simulink model "uz_ParameterID6ph"  (R2021b)
settings: Solver=FixedStepDiscrete  StartTime=0.0  StopTime=160  FixedStep=0.000005  RelTol=1e-3  EnableMultiTasking=on
model workspace (MATLAB code in the model file):
  | cmdLim = Simulink.Parameter;
  | cmdLim.Value = 15;
  | cmdLim.Description = 'Limit for controlling the maximum surface command angle.';
  | cmdLim.Min = 0;
  | cmdLim.Max = 90;
  | cmdLim.DocUnits = 'deg';
  | 
  | dispGain = Simulink.Parameter;
  | dispGain.Value = 0.75;
  | dispGain.Description = 'Gain applied to the displacement error.';
  | dispGain.Min = 0;
  | dispGain.Max = [];
  | dispGain.DocUnits = 'deg/sec/deg';
  | 
  | dispLim = Simulink.Parameter;
  | dispLim.Value = 30;
  | dispLim.Description = 'Limit for controlling the maximum commanded angle.';
  | dispLim.Min = 0;
  | dispLim.Max = 180;
  | dispLim.DocUnits = 'deg';
  | 
  | intGain = Simulink.Parameter;
  | intGain.Value = 0.5;
  | intGain.Description = 'Gain applied to the integral error.';
  | intGain.Min = 0;
  | intGain.Max = [];
  | intGain.DocUnits = 'deg/sec/deg/sec';
  | 
  | intLim = Simulink.Parameter;
  | intLim.Value = 5;
  | intLim.Description = 'Limit for controlling the maximum commanded angle.';
  | intLim.Min = 0;
  | intLim.Max = 90;
  | intLim.DocUnits = 'deg';
  | 
  | rateGain = Simulink.Parameter;
  | rateGain.Value = 2;
  | rateGain.Description = 'Gain applied to the rate error.';
  | rateGain.Min = 0;
  | rateGain.Max = [];
  | rateGain.DocUnits = 'deg/deg/sec';
  | 
  | rateLim = Simulink.Parameter;
  | rateLim.Value = 6;
  | rateLim.Description = 'Limit for controlling the maximum commanded angle.';
  | rateLim.Min = 0;
  | rateLim.Max = 180;
  | rateLim.DocUnits = 'deg/sec';
  | 
  | hdgGain = Simulink.Parameter;
  | hdgGain.Value = 0.015;
values from neighbouring files (symbols this model uses):
  c = 2/6*cat(1,tl1,tl2,tl3,tl4,tl5,tl6)    [Parameter_Init_Buehler_201_6ph.m]
  d_d_TMS = 0.005    [Parameter_Init_Buehler_201.m]
  d_f_hardware = 200000    [Parameter_Init_Buehler_201.m]
  d_f_states = 20000    [Parameter_Init_Buehler_201.m]
  d_i_max = 15    [Parameter_Init_Buehler_201.m]
  d_i_min = -d_i_max    (= -15)    [Parameter_Init_Buehler_201.m]
  d_I_n = 8    [Parameter_Init_Buehler_201.m]
  d_J_Coupling_M_E = 2e-6    (= 2e-06)    [Parameter_Init_Buehler_201.m]
  d_J_Coupling_M_Ms = 2e-20    [Parameter_Init_Buehler_201.m]
  d_J_Ms_L = d_J_Ms_M    (= 1.26363648e-05)    [Parameter_Init_Buehler_201.m]
  d_J_Ms_M = 0.5*0.5*((0.5*d_d_Ms)^4)*3.14*d_l_Ms*d_rho_Ms    (= 1.26363648e-05)    [Parameter_Init_Buehler_201.m]
  d_Ki_id = 162.47    [Parameter_Init_Buehler_201.m]
  d_Ki_iq = 162.47    [Parameter_Init_Buehler_201.m]
  d_Ki_n = 1.982    [Parameter_Init_Buehler_201.m]
  d_Kp_id = 0.369    [Parameter_Init_Buehler_201.m]
  d_Kp_iq = 0.369    [Parameter_Init_Buehler_201.m]
  d_Kp_n = 0.198    [Parameter_Init_Buehler_201.m]
  d_L_d = 0.00031    [Parameter_Init_Buehler_201.m]
  d_L_q = 0.00033    [Parameter_Init_Buehler_201.m]
  d_n_n = 3200    [Parameter_Init_Buehler_201.m]
  d_p = 4    [Parameter_Init_Buehler_201.m]
  d_psi_pm = 0.0075    [Parameter_Init_Buehler_201.m]
  d_R_ph = d_R_ph_ph/2    (= 0.089)    [Parameter_Init_Buehler_201.m]
  d_y_max = 10    [Parameter_Init_Buehler_201.m]
  d_y_min = -d_y_max    (= -10)    [Parameter_Init_Buehler_201.m]
  V_DC = 24    [Parameter_Init_Buehler_201.m]
undefined symbols (not defined in the file or in its folder): i_dq, i_dq_ref, n_ref, ts_ps, V_abc, v_dq
libraries: fl_lib x66, nesl_utility x51, ee_lib x38, simulink x14, spsTriangleGeneratorLib x3, spsabctodq0Lib x2, spsAlphaBetaZerotodq0Lib x2, spsdq0toabcLib x1
(part 3 of 6)

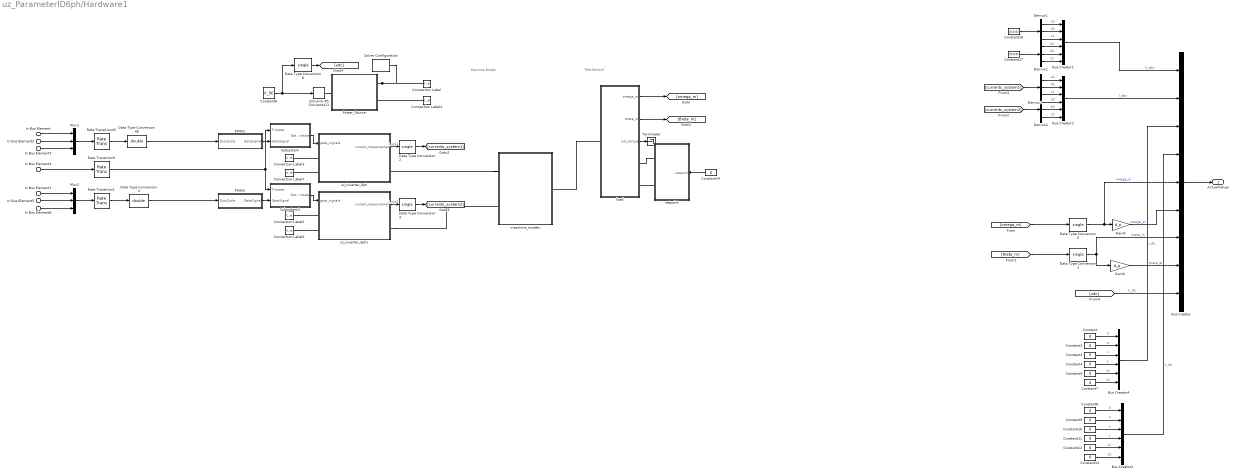
== system uz_ParameterID6ph/Hardware1 ==
  note: Mechanical
  note: Machine Model
  In Bus Element : Inport  PortName=ElectricalID_output  Element=PWM_Switch_a1
  In Bus Element2 : Inport  PortName=ElectricalID_output  Element=PWM_Switch_b1
  In Bus Element3 : Inport  PortName=ElectricalID_output  Element=PWM_Switch_c1
  In Bus Element4 : Inport  PortName=ElectricalID_output  Element=enable_TriState
  In Bus Element1 : Inport  PortName=ElectricalID_output  Element=PWM_Switch_a2
  In Bus Element5 : Inport  PortName=ElectricalID_output  Element=PWM_Switch_b2
  In Bus Element6 : Inport  PortName=ElectricalID_output  Element=PWM_Switch_c2
  Bus Creator : BusCreator  Inputs=9  OutDataTypeStr=Bus: uz_ParaID6ph_ActualValues_t
  Bus Creator1 : BusCreator  Inputs=6  OutDataTypeStr=Bus: uz_6ph_abc_t
  Bus Creator2 : BusCreator  Inputs=6  OutDataTypeStr=Bus: uz_6ph_abc_t
  Bus Creator3 : BusCreator  Inputs=6  OutDataTypeStr=Bus: uz_6ph_dq_t
  Bus Creator4 : BusCreator  Inputs=6  OutDataTypeStr=Bus: uz_6ph_dq_t
  Connection Label : ConnectionLabel  Label=udc_plus
  Connection Label2 : ConnectionLabel  Label=udc_plus
  Connection Label3 : ConnectionLabel  Label=udc_plus
  Connection Label4 : ConnectionLabel  Label=udc_minus
  Connection Label6 : ConnectionLabel  Label=udc_minus
  Connection Label7 : ConnectionLabel  Label=udc_minus
  Constant{,2..5,7..13} (12 alike) : Constant  Value=0  OutDataTypeStr=single  SampleTime=-1
  Constant14 : Constant  Value=0  OutDataTypeStr=double  SampleTime=ts_ps
  Constant16 : Constant  Value=[0;0;0]  OutDataTypeStr=single  SampleTime=-1
  Constant17 : Constant  Value=[0;0;0]  OutDataTypeStr=single  SampleTime=-1
  Constant6 : Constant  Value=V_DC  SampleTime=ts_ps
  Data Type Conversion{1..3,5..6} (5 alike) : DataTypeConversion  OutDataTypeStr=single
  Data Type Conversion4 : DataTypeConversion  OutDataTypeStr=double
  Data Type Conversion48 : DataTypeConversion  OutDataTypeStr=double
  Demux{1..4} (4 alike) : Demux  Outputs=3
  Gain6 : Gain  Gain=d_p  OutDataTypeStr=single
  Gain9 : Gain  Gain=d_p  OutDataTypeStr=single
  Mux1 : Mux  Inputs=3
  Mux2 : Mux  Inputs=3
  PWM1 : Subsystem
  PWM2 : Subsystem
  Power_Source : Subsystem
  Rate Transition1 : RateTransition  OutPortSampleTime=1/d_f_hardware
  Rate Transition45 : RateTransition  OutPortSampleTime=1/d_f_hardware
  Rate Transition9 : RateTransition  OutPortSampleTime=1/d_f_hardware
  Simulink-PS Converter11 : nesl_utility/Simulink-PS Converter  PhysicalDomain=network_engine_domain  SubClassName=ps_input  LeftPortType=input  RightPortType=output  PseudoPeriodic=off  Frequencies=[]  NoiseDistribution=none  NoiseParameters=[]  Unit=1  AffineConversion=off  FilteringAndDerivatives=provide  SimscapeFilterOrder=1  InputFilterTimeConstant=0.001  UdotUserProvided=0
      settings: SourceProductBaseCode=PW,SS
  Solver Configuration : nesl_utility/Solver Configuration  PhysicalDomain=network_engine_domain  SubClassName=solver  LeftPortType=input  RightPortType=generic  Tones=[]  Harmonics=[]  SimulateNoise=off  Profile=off  UseLocalSampling=off  EnableSwitchedLinearOptims=on  FrequencyDomain=off  UseCCode=off  RelTol=0.001  AbsTol=1e-06  MinStep=1e-09  ToWorkspace=off  RevertToSquareIcSolve=off  NumHomotopyIterations=100  PhasorMode=off  PhasorModeNumHarmonics=1  DoDC=off  ResidualTolerance=1e-09  UseLocalSolver=on  LocalSolverChoice=NE_BACKWARD_EULER_ADVANCER  LocalSolverSampleTime=1e-8  DoFixedCost=on  MaxNonlinIter=3  MaxModeIter=2  ComputeImpulses=off  ImpulseIterations=2  LinearAlgebra=auto  EquationFormulation=NE_TIME_EF  DelaysMemoryBudget=1024  AutomaticFiltering=on  FilteringTimeConstant=0.001  PartitionStorageMethod=AS_NEEDED  PartitionMemoryBudget=1024  PartitionMethod=ROBUST
      settings: SourceProductBaseCode=PW,SS
  Subsystem : Subsystem
  Subsystem1 : Subsystem
  Terminator : Terminator
  load : Subsystem
  maschine_models : Subsystem  Variant=on  VariantControlMode=label  LabelModeActiveChoice=neutral_isolated_vsd
  setpoint : Subsystem  Variant=on  VariantControlMode=label  LabelModeActiveChoice=torque_load
  uz_inverter_3ph : Subsystem
  uz_inverter_3ph1 : Subsystem
  ActualValues : Outport
  wires:
  Mux1/1 -> Rate Transition45/1
  Data Type Conversion1/1 -> Bus Creator/7, Gain6/1  "theta_m"
  Gain9/1 -> Bus Creator/6  "omega_el"
  Bus Creator/1 -> ActualValues/1
  Data Type Conversion5/1 -> Gain9/1, Bus Creator/5  "omega_m"
  In Bus Element4/1 -> Rate Transition9/1
  In Bus Element/1 -> Mux1/1
  In Bus Element3/1 -> Mux1/3
  In Bus Element2/1 -> Mux1/2
  Rate Transition45/1 -> Data Type Conversion48/1
  Constant/1 -> Bus Creator4/1  "d"
  Bus Creator4/1 -> Bus Creator/3  "i_dq"
  Bus Creator2/1 -> Bus Creator/2  "I_abc"
  Bus Creator1/1 -> Bus Creator/1  "V_abc"
  Gain6/1 -> Bus Creator/8  "theta_el"
  uz_inverter_3ph1/1(current_measurement) -> Data Type Conversion3/1  "i_sys2"
  uz_inverter_3ph/1(current_measurement) -> Data Type Conversion2/1  "i_sys1"
  Subsystem1/1(GateTristate) -> uz_inverter_3ph1/1(gate_signals)
  Constant6/1 -> Simulink-PS Converter11/1, Data Type Conversion6/1
  PWM1/1(GateSignal) -> Subsystem/2(GateSignal)
  Subsystem/1(GateTristate) -> uz_inverter_3ph/1(gate_signals)
  PWM2/1(GateSignal) -> Subsystem1/2(GateSignal)
  load/1(omega_m) -> [omega_m]
  load/2(theta_m) -> [theta_m]
  [omega_m] -> Data Type Conversion5/1
  [theta_m] -> Data Type Conversion1/1
  [udc] -> Bus Creator/9  "V_DC"
  Demux1/3 -> Bus Creator1/3  "c1"
  Demux1/2 -> Bus Creator1/2  "b1"
  Demux1/1 -> Bus Creator1/1  "a1"
  Demux2/1 -> Bus Creator1/4  "a2"
  Demux2/2 -> Bus Creator1/5  "b2"
  Demux2/3 -> Bus Creator1/6  "c2"
  Demux4/3 -> Bus Creator2/6  "c2"
  Demux4/2 -> Bus Creator2/5  "b2"
  Demux4/1 -> Bus Creator2/4  "a2"
  Demux3/1 -> Bus Creator2/1  "a1"
  Demux3/2 -> Bus Creator2/2  "b1"
  Demux3/3 -> Bus Creator2/3  "c1"
  [currents_system1] -> Demux3/1
  [currents_system2] -> Demux4/1
  Constant7/1 -> Bus Creator4/6  "z2"
  Constant5/1 -> Bus Creator4/5  "z1"
  Constant4/1 -> Bus Creator4/4  "y"
  Constant3/1 -> Bus Creator4/3  "x"
  Constant2/1 -> Bus Creator4/2  "q"
  Constant9/1 -> Bus Creator3/2  "q"
  Constant10/1 -> Bus Creator3/3  "x"
  Constant11/1 -> Bus Creator3/4  "y"
  Constant12/1 -> Bus Creator3/5  "z1"
  Constant13/1 -> Bus Creator3/6  "z2"
  Bus Creator3/1 -> Bus Creator/4  "v_dq"
  Constant8/1 -> Bus Creator3/1  "d"
  Data Type Conversion48/1 -> PWM1/1(DutyCycle)
  Rate Transition9/1 -> Subsystem1/1(Tristate), Subsystem/1(Tristate)
  Constant16/1 -> Demux1/1
  Constant17/1 -> Demux2/1
  Data Type Conversion2/1 -> [currents_system1]
  Data Type Conversion3/1 -> [currents_system2]
  Constant14/1 -> setpoint/1(setpoint)
  load/3(out_torque) -> Terminator/1
  Rate Transition1/1 -> Data Type Conversion4/1
  In Bus Element5/1 -> Mux2/2
  In Bus Element6/1 -> Mux2/3
  In Bus Element1/1 -> Mux2/1
  Mux2/1 -> Rate Transition1/1
  Data Type Conversion4/1 -> PWM2/1(DutyCycle)
  Data Type Conversion6/1 -> [udc]
  connections:
  Power_Source/RConn1 -- Solver Configuration/RConn1 -- Connection Label/LConn1
  Simulink-PS Converter11/RConn1 -- Power_Source/LConn1
  Connection Label2/LConn1 -- uz_inverter_3ph1/LConn1
  Connection Label3/LConn1 -- uz_inverter_3ph/LConn1
  Connection Label6/LConn1 -- uz_inverter_3ph1/LConn2
  Connection Label7/LConn1 -- uz_inverter_3ph/LConn2
  Connection Label4/LConn1 -- Power_Source/RConn2
  maschine_models/LConn1 -- uz_inverter_3ph/RConn1
  setpoint/RConn2 -- load/RConn2
  load/LConn1 -- maschine_models/RConn1
  uz_inverter_3ph1/RConn1 -- maschine_models/LConn2
  setpoint/RConn1 -- load/RConn1

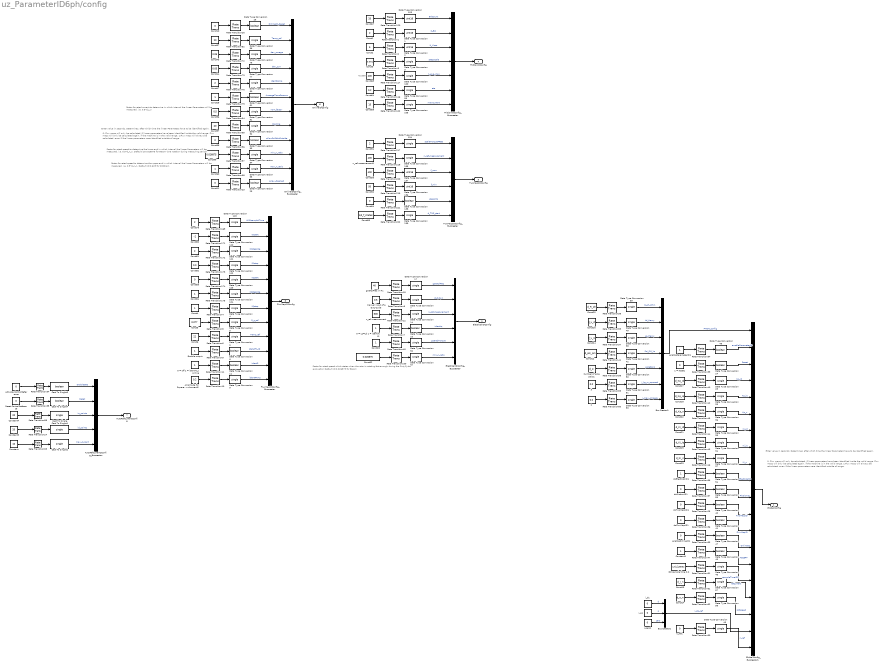
== system uz_ParameterID6ph/config ==
  note: %1000
  note: Factor for rated speed,to determine the upper end in which interval the linear Parameters will
      | be measured. i.e. 0,5*d_n_n.
      | Default ist 0.625 for 2000rpm
  note: 0: Flux maps will only be calculated, if linear parameters have been identified inside the valid range.
      |     Flux maps will only be calculated again, if the machine is in the valid range.
      | 1:Flux maps will always be calculated, even if the linear parameters were identified outside of range.
  note: Enter value in seconds. Determines, after which time the linear Parameters have to be identified again.
  note: Factor for rated current,to determine in which interval the linear Parameters will
      | be measured. i.e. 0,5*d_I_n
  note: Factor for rated speed,to determine the lower end in which interval the linear Parameters will
      | be measured. i.e. 0,5*d_n_n.
      | Default ist 0.026875 for 86rpm (one rotation during measuring period)
  note: Factor for rated speed,which states when the rotor is rotating fast enough during the DutyCycle evaluation
      | Default ist 0.026875 for 86rpm
  note: 0: Flux maps will only be calculated, if linear parameters have been identified inside the valid range.
      |     Flux maps will only be calculated again, if the machine is in the valid range.
      | 1:Flux maps will always be calculated, even if the linear parameters were identified outside of range.
  note: Enter value in seconds. Determines, after which time the linear Parameters have to be identified again.
  "0 = Lq=Ld 1 = identify Lq " : Constant
  0 = off 1 = ident R_s online : Constant
  1 = reset1 : Constant  Value=0
  2 : Constant  Value=0.0
  3 : Constant  Value=0.0
  Activate ControlReference : Constant  Value=0  OutDataTypeStr=boolean
  Amplitude for SquareWave signal in d-current2 : Constant  Value=0.2
  AutoRefCurrentsConfig_Buscreator : BusCreator  Inputs=5  OutDataTypeStr=Bus: uz_ParaID_AutoRefCurrentsConfig_t
  Bus Creator1 : BusCreator  Inputs=7  OutDataTypeStr=Bus: uz_PMSM_t
  Bus Creator2 : BusCreator  Inputs=3  OutDataTypeStr=Bus: uz_3ph_dq_t
  Cast To Single : DataTypeConversion  OutDataTypeStr=single
  Cast To Single1 : DataTypeConversion  OutDataTypeStr=single
  Cast To Single2 : DataTypeConversion  OutDataTypeStr=single
  Cast To Single3 : DataTypeConversion  OutDataTypeStr=boolean
  Cast To Single4 : DataTypeConversion  OutDataTypeStr=boolean
  Const{1,47,78,81,91} (5 alike) : Constant  Value=2
  Const{10..11,58,83,94} (5 alike) : Constant  Value=0
  Const12 : Constant  Value=d_psi_pm
  Const13 : Constant  Value=d_I_n
  Const14 : Constant  Value=d_n_n
  Const16 : Constant  Value=d_L_d
  Const17 : Constant  Value=d_Kp_id
  Const18 : Constant  Value=d_Kp_iq
  Const19 : Constant  Value=d_Ki_iq
  Const2 : Constant  Value=5
  Const{4,20,28,60,84} (5 alike) : Constant
  Const21 : Constant  Value=d_Ki_id
  Const22 : Constant  Value=d_Kp_n
  Const23 : Constant  Value=d_Ki_n
  Const24 : Constant  Value=d_L_q
  Const25 : Constant  Value=d_R_ph
  Const3 : Constant  Value=0.001
  Const37 : Constant  Value=20
  Const43 : Constant  Value=0.05
  Const44 : Constant  Value=0.05
  Const5 : Constant  Value=0.077
  Const56 : Constant  Value=0.5
  Const57 : Constant  Value=20
  Const59 : Constant  Value=0.026875
  Const6 : Constant  Value=22
  Const62 : Constant  Value=0.026875
  Const64 : Constant  Value=0.2
  Const65 : Constant  Value=200
  Const67 : Constant  Value=20
  Const69 : Constant  Value=15
  Const80 : Constant  Value=-2
  Const82 : Constant  Value=0.0
  Const92 : Constant  Value=50
  Const93 : Constant  Value=400
  Const95 : Constant  Value=1/d_f_states
  Constant : Constant  Value=10
  Constant1 : Constant
  Constant3 : Constant  Value=20
  Constant4 : Constant  Value=20
  Data Type Conversion{1..2,103,136..137} (5 alike) : DataTypeConversion  OutDataTypeStr=uint16
  Data Type Conversion{8,10..11,23..24,26,40..41,43,47..48,54..55,61,93,138} (16 alike) : DataTypeConversion  OutDataTypeStr=boolean
  Data Type Conversion{3..7,9,14,17,25,33..39,42,45..46,49..53,56..58,76..77,80,91..92,94..95,97,99..100,105,118,120..124,134..135,139} (47 alike) : DataTypeConversion  OutDataTypeStr=single
  ElectricalIDConfig_Buscreater : BusCreator  Inputs=6  OutDataTypeStr=Bus: uz_ParaID_ElectricalIDConfig_t
  Enable output : Constant
  FluxMapIDConfig_Buscreater : BusCreator  Inputs=12  OutDataTypeStr=Bus: uz_ParaID_FluxMapIDConfig_t
  FrictionIDConfig_Buscreater : BusCreator  Inputs=7  OutDataTypeStr=Bus: uz_ParaID_FrictionIDConfig_t
  GlobalConfig_Buscreator1 : BusCreator  Inputs=20  OutDataTypeStr=Bus: uz_ParaID_GlobalConfig_t
  ISR sample time 0.2 : Constant  Value=1/d_f_states
  Number of pole pairs1 : Constant  Value=d_p
  OnlineIDConfig_Buscreater : BusCreator  Inputs=12  OutDataTypeStr=Bus: uz_ParaID_OnlineIDConfig_t
  Rate Transition{1..12,18,23..26,33..48,50..62,72..73,76,79,88,94..98,100,116..117,120,122,169,171..175,217..222} (73 alike) : RateTransition  OutPortSampleTime=1/d_f_states
  Reset ControlReference : Constant  Value=0  OutDataTypeStr=boolean
  TwoMassIDConfig_Buscreater : BusCreator  Inputs=6  OutDataTypeStr=Bus: uz_ParaID_TwoMassIDConfig_t
  doElectricalID1 : Constant
  doFluxMapID1 : Constant  Value=0
  doFrictionID1 : Constant  Value=0
  doTwoMassID1 : Constant  Value=0
  enableOnlineID1 : Constant  Value=0
  enableParameterID1 : Constant
  goertzlFreq in Hz : Constant  Value=40
  i_d1 : Constant  Value=0  OutDataTypeStr=single
  i_q1 : Constant  Value=0  OutDataTypeStr=single
  i_zero1 : Constant  Value=0  OutDataTypeStr=single
  manual input of a DutyCycle : Constant  Value=0.5
  n_ref measurement : Constant  Value=500
  n_ref measurement1 : Constant  Value=400
  n_ref1 : Constant  Value=0
  GlobalConfig : Outport
  ElectricalIDConfig : Outport  Port=2
  FluxMapIDConfig : Outport  Port=3
  FrictionIDConfig : Outport  Port=4
  TwoMassIDConfig : Outport  Port=5
  OnlineIDConfig : Outport  Port=6
  AutoRefCurrentsconfig : Outport  Port=7
  wires:
  Data Type Conversion1/1 -> FrictionIDConfig_Buscreater/2  "N_Brk"
  Data Type Conversion99/1 -> FrictionIDConfig_Buscreater/6  "eta"
  Data Type Conversion2/1 -> FrictionIDConfig_Buscreater/3  "N_Visco"
  Data Type Conversion103/1 -> FrictionIDConfig_Buscreater/1  "BrkCount"
  Data Type Conversion105/1 -> FrictionIDConfig_Buscreater/7  "maxCurrent"
  Data Type Conversion100/1 -> FrictionIDConfig_Buscreater/5  "n_eva_max"
  Data Type Conversion3/1 -> FrictionIDConfig_Buscreater/4  "StepScale"
  FrictionIDConfig_Buscreater/1 -> FrictionIDConfig/1
  Rate Transition120/1 -> Data Type Conversion103/1
  Const67/1 -> Rate Transition120/1
  Const1/1 -> Rate Transition1/1
  Rate Transition1/1 -> Data Type Conversion1/1
  Const2/1 -> Rate Transition2/1
  Rate Transition2/1 -> Data Type Conversion2/1
  Const3/1 -> Rate Transition3/1
  Rate Transition3/1 -> Data Type Conversion3/1
  Const65/1 -> Rate Transition117/1
  Const64/1 -> Rate Transition116/1
  Rate Transition116/1 -> Data Type Conversion99/1
  Rate Transition117/1 -> Data Type Conversion100/1
  Const69/1 -> Rate Transition122/1
  Rate Transition122/1 -> Data Type Conversion105/1
  TwoMassIDConfig_Buscreater/1 -> TwoMassIDConfig/1
  Const91/1 -> Rate Transition217/1
  Rate Transition217/1 -> Data Type Conversion134/1
  Data Type Conversion134/1 -> TwoMassIDConfig_Buscreater/1  "ScaleTorquePRBS"
  Rate Transition218/1 -> Data Type Conversion135/1
  n_ref measurement1/1 -> Rate Transition218/1
  Data Type Conversion135/1 -> TwoMassIDConfig_Buscreater/2  "n_ref_measurement"
  Rate Transition219/1 -> Data Type Conversion136/1
  Const93/1 -> Rate Transition220/1
  Const92/1 -> Rate Transition219/1
  Rate Transition220/1 -> Data Type Conversion137/1
  Data Type Conversion137/1 -> TwoMassIDConfig_Buscreater/3  "f_max"
  Data Type Conversion136/1 -> TwoMassIDConfig_Buscreater/4  "f_min"
  Rate Transition221/1 -> Data Type Conversion138/1
  Rate Transition222/1 -> Data Type Conversion139/1
  Const94/1 -> Rate Transition221/1
  Const95/1 -> Rate Transition222/1
  Data Type Conversion138/1 -> TwoMassIDConfig_Buscreater/5  "UseLbMq"
  Data Type Conversion139/1 -> TwoMassIDConfig_Buscreater/6  "d_TMS_start"
  FluxMapIDConfig_Buscreater/1 -> FluxMapIDConfig/1
  Rate Transition172/1 -> Data Type Conversion121/1
  Const80/1 -> Rate Transition171/1
  Const84/1 -> Rate Transition175/1
  Rate Transition175/1 -> Data Type Conversion124/1
  Rate Transition171/1 -> Data Type Conversion120/1
  Rate Transition174/1 -> Data Type Conversion123/1
  Const78/1 -> Rate Transition169/1
  Const82/1 -> Rate Transition173/1
  Const81/1 -> Rate Transition172/1
  Rate Transition169/1 -> Data Type Conversion118/1
  Rate Transition173/1 -> Data Type Conversion122/1
  Const83/1 -> Rate Transition174/1
  Data Type Conversion118/1 -> FluxMapIDConfig_Buscreater/1  "AMMsampleTime"
  Data Type Conversion120/1 -> FluxMapIDConfig_Buscreater/2  "IDstart"
  Rate Transition5/1 -> Data Type Conversion5/1
  Rate Transition6/1 -> Data Type Conversion6/1
  Const6/1 -> Rate Transition6/1
  Const4/1 -> Rate Transition4/1
  Const5/1 -> Rate Transition5/1
  Rate Transition4/1 -> Data Type Conversion4/1
  Data Type Conversion121/1 -> FluxMapIDConfig_Buscreater/3  "IDstepsize"
  Data Type Conversion122/1 -> FluxMapIDConfig_Buscreater/4  "IDstop"
  Data Type Conversion123/1 -> FluxMapIDConfig_Buscreater/5  "IQstart"
  Data Type Conversion124/1 -> FluxMapIDConfig_Buscreater/6  "IQstepsize"
  Data Type Conversion4/1 -> FluxMapIDConfig_Buscreater/7  "IQstop"
  Data Type Conversion5/1 -> FluxMapIDConfig_Buscreater/8  "R_s_ref"
  Data Type Conversion6/1 -> FluxMapIDConfig_Buscreater/9  "Temp_ref"
  ElectricalIDConfig_Buscreater/1 -> ElectricalIDConfig/1
  OnlineIDConfig_Buscreater/1 -> OnlineIDConfig/1
  Const37/1 -> Rate Transition52/1
  Rate Transition52/1 -> Data Type Conversion56/1
  Data Type Conversion56/1 -> OnlineIDConfig_Buscreater/2  "Temp_ref"
  Data Type Conversion77/1 -> OnlineIDConfig_Buscreater/4  "dev_curr"
  Data Type Conversion76/1 -> OnlineIDConfig_Buscreater/3  "dev_omega"
  Const44/1 -> Rate Transition73/1
  Const43/1 -> Rate Transition72/1
  Rate Transition72/1 -> Data Type Conversion76/1
  Const47/1 -> Rate Transition76/1
  Rate Transition73/1 -> Data Type Conversion77/1
  Rate Transition76/1 -> Data Type Conversion80/1
  Data Type Conversion80/1 -> OnlineIDConfig_Buscreater/5  "identRAmp"
  Data Type Conversion61/1 -> OnlineIDConfig_Buscreater/6  "AverageTransParams"
  Const28/1 -> Rate Transition79/1
  Rate Transition79/1 -> Data Type Conversion61/1
  Const56/1 -> Rate Transition94/1
  Data Type Conversion93/1 -> OnlineIDConfig_Buscreater/9  "allowPsiCalcOutside"
  Rate Transition94/1 -> Data Type Conversion91/1
  Data Type Conversion95/1 -> OnlineIDConfig_Buscreater/11  "max_n_ratio"
  Const58/1 -> Rate Transition96/1
  Const57/1 -> Rate Transition95/1
  Data Type Conversion91/1 -> OnlineIDConfig_Buscreater/7  "nom_factor"
  Rate Transition98/1 -> Data Type Conversion95/1
  Data Type Conversion92/1 -> OnlineIDConfig_Buscreater/8  "Rs_time"
  Rate Transition96/1 -> Data Type Conversion93/1
  Const59/1 -> Rate Transition97/1
  Rate Transition97/1 -> Data Type Conversion94/1
  Const60/1 -> Rate Transition98/1
  Data Type Conversion94/1 -> OnlineIDConfig_Buscreater/10  "min_n_ratio"
  Rate Transition95/1 -> Data Type Conversion92/1
  Rate Transition26/1 -> Data Type Conversion26/1
  Data Type Conversion26/1 -> OnlineIDConfig_Buscreater/1  "OnlineID_Reset"
  Const10/1 -> Rate Transition26/1
  Data Type Conversion11/1 -> FluxMapIDConfig_Buscreater/11  "identR"
  0 = off 1 = ident R_s online/1 -> Rate Transition11/1
  Rate Transition10/1 -> Data Type Conversion9/1
  Amplitude for SquareWave signal in d-current2/1 -> Rate Transition10/1
  Data Type Conversion9/1 -> FluxMapIDConfig_Buscreater/12  "identRAmp"
  Rate Transition11/1 -> Data Type Conversion11/1
  Data Type Conversion8/1 -> FluxMapIDConfig_Buscreater/10  "start_FM_ID"
  Rate Transition9/1 -> Data Type Conversion8/1
  Enable output/1 -> Rate Transition9/1
  Rate Transition23/1 -> Data Type Conversion23/1
  Const11/1 -> Rate Transition23/1
  Data Type Conversion23/1 -> OnlineIDConfig_Buscreater/12  "array_cleaned"
  Constant4/1 -> Rate Transition88/1
  Rate Transition88/1 -> Cast To Single/1
  Rate Transition24/1 -> Cast To Single1/1
  Constant3/1 -> Rate Transition24/1
  Rate Transition33/1 -> Cast To Single2/1
  Constant/1 -> Rate Transition33/1
  Rate Transition34/1 -> Cast To Single3/1
  Cast To Single3/1 -> AutoRefCurrentsConfig_Buscreator/1  "enableCRS"
  Activate ControlReference/1 -> Rate Transition34/1
  Rate Transition35/1 -> Cast To Single4/1
  Reset ControlReference/1 -> Rate Transition35/1
  Cast To Single4/1 -> AutoRefCurrentsConfig_Buscreator/2  "Reset"
  Cast To Single/1 -> AutoRefCurrentsConfig_Buscreator/3  "iq_points"
  Cast To Single1/1 -> AutoRefCurrentsConfig_Buscreator/4  "id_points"
  Cast To Single2/1 -> AutoRefCurrentsConfig_Buscreator/5  "max_current"
  AutoRefCurrentsConfig_Buscreator/1 -> AutoRefCurrentsconfig/1
  Rate Transition18/1 -> Data Type Conversion17/1
  Data Type Conversion17/1 -> ElectricalIDConfig_Buscreater/1  "goertzlFreq"
  goertzlFreq in Hz/1 -> Rate Transition18/1
  Rate Transition8/1 -> Data Type Conversion7/1
  Const20/1 -> Rate Transition48/1
  Data Type Conversion14/1 -> ElectricalIDConfig_Buscreater/3  "n_ref_measurement"
  manual input of a DutyCycle/1 -> Rate Transition8/1
  "0 = Lq=Ld 1 = identify Lq "/1 -> Rate Transition7/1
  Const62/1 -> Rate Transition100/1
  n_ref measurement/1 -> Rate Transition12/1
  Data Type Conversion7/1 -> ElectricalIDConfig_Buscreater/2  "dutyCyc"
  Data Type Conversion97/1 -> ElectricalIDConfig_Buscreater/6  "min_n_ratio"
  Rate Transition7/1 -> Data Type Conversion10/1
  Rate Transition48/1 -> Data Type Conversion52/1
  Rate Transition12/1 -> Data Type Conversion14/1
  Data Type Conversion52/1 -> ElectricalIDConfig_Buscreater/5  "goertzlTorque"
  Data Type Conversion10/1 -> ElectricalIDConfig_Buscreater/4  "identLq"
  Rate Transition100/1 -> Data Type Conversion97/1
  Rate Transition25/1 -> Data Type Conversion40/1
  Rate Transition62/1 -> Data Type Conversion58/1
  Const25/1 -> Rate Transition38/1
  Rate Transition51/1 -> Data Type Conversion46/1
  Data Type Conversion24/1 -> GlobalConfig_Buscreator1/3  "Reset"
  Data Type Conversion45/1 -> GlobalConfig_Buscreator1/20  "n_ref"
  ISR sample time 0.2/1 -> Rate Transition51/1
  Bus Creator2/1 -> GlobalConfig_Buscreator1/19  "i_dq_ref"
  Rate Transition50/1 -> Data Type Conversion45/1
  n_ref1/1 -> Rate Transition50/1
  Rate Transition55/1 -> Data Type Conversion49/1
  Rate Transition61/1 -> Data Type Conversion57/1
  Const12/1 -> Rate Transition41/1
  Rate Transition59/1 -> Data Type Conversion51/1
  3/1 -> Rate Transition59/1
  Rate Transition38/1 -> Data Type Conversion39/1
  Rate Transition46/1 -> Data Type Conversion37/1
  Const24/1 -> Rate Transition37/1
  Data Type Conversion38/1 -> Bus Creator1/3  "Lq_Henry"
  Data Type Conversion34/1 -> GlobalConfig_Buscreator1/8  "Ki_iq"
  Const14/1 -> Rate Transition62/1
  Rate Transition53/1 -> Data Type Conversion47/1
  Rate Transition41/1 -> Data Type Conversion42/1
  Bus Creator1/1 -> GlobalConfig_Buscreator1/1  "PMSM_config"
  Data Type Conversion42/1 -> Bus Creator1/4  "Psi_PM_Vs"
  Data Type Conversion41/1 -> GlobalConfig_Buscreator1/13  "FluxMapID"
  Rate Transition56/1 -> Data Type Conversion54/1
  Const13/1 -> Rate Transition61/1
  Data Type Conversion40/1 -> GlobalConfig_Buscreator1/12  "TwoMassID"
  Constant1/1 -> Rate Transition47/1
  Rate Transition47/1 -> Data Type Conversion43/1
  Data Type Conversion37/1 -> GlobalConfig_Buscreator1/9  "Ki_n"
  Data Type Conversion53/1 -> Bus Creator1/7  "I_max_Ampere"
  doTwoMassID1/1 -> Rate Transition25/1
  Data Type Conversion35/1 -> GlobalConfig_Buscreator1/7  "Ki_id"
  Data Type Conversion54/1 -> GlobalConfig_Buscreator1/10  "ElectricalID"
  Rate Transition45/1 -> Data Type Conversion36/1
  doFrictionID1/1 -> Rate Transition57/1
  Rate Transition36/1 -> Data Type Conversion41/1
  doElectricalID1/1 -> Rate Transition56/1
  Data Type Conversion55/1 -> GlobalConfig_Buscreator1/11  "FrictionID"
  Rate Transition43/1 -> Data Type Conversion34/1
  Rate Transition57/1 -> Data Type Conversion55/1
  Rate Transition39/1 -> Data Type Conversion24/1
  Const18/1 -> Rate Transition42/1
  Data Type Conversion47/1 -> GlobalConfig_Buscreator1/14  "OnlineID"
  Const21/1 -> Rate Transition44/1
  i_q1/1 -> Bus Creator2/2  "q"
  enableParameterID1/1 -> Rate Transition54/1
  Rate Transition44/1 -> Data Type Conversion35/1
  Const19/1 -> Rate Transition43/1
  Data Type Conversion49/1 -> Bus Creator1/2  "Ld_Henry"
  Number of pole pairs1/1 -> Rate Transition58/1
  Data Type Conversion50/1 -> Bus Creator1/5  "polePairs"
  Data Type Conversion46/1 -> GlobalConfig_Buscreator1/16  "sampleTimeISR"
  Rate Transition54/1 -> Data Type Conversion48/1
  Rate Transition58/1 -> Data Type Conversion50/1
  Data Type Conversion51/1 -> Bus Creator1/6  "J_kg_m_squared"
  Data Type Conversion58/1 -> GlobalConfig_Buscreator1/18  "ratSpeed"
  Data Type Conversion57/1 -> GlobalConfig_Buscreator1/17  "ratCurrent"
  Rate Transition42/1 -> Data Type Conversion33/1
  Data Type Conversion43/1 -> GlobalConfig_Buscreator1/15  "ACCEPT"
  i_d1/1 -> Bus Creator2/1  "d"
  Data Type Conversion48/1 -> GlobalConfig_Buscreator1/2  "enableParameterID"
  Data Type Conversion39/1 -> Bus Creator1/1  "R_ph_Ohm"
  GlobalConfig_Buscreator1/1 -> GlobalConfig/1
  i_zero1/1 -> Bus Creator2/3  "zero"
  Rate Transition37/1 -> Data Type Conversion38/1
  1 = reset1/1 -> Rate Transition39/1
  Data Type Conversion25/1 -> GlobalConfig_Buscreator1/4  "Kp_id"
  doFluxMapID1/1 -> Rate Transition36/1
  Rate Transition40/1 -> Data Type Conversion25/1
  Const16/1 -> Rate Transition55/1
  Data Type Conversion33/1 -> GlobalConfig_Buscreator1/5  "Kp_iq"
  Data Type Conversion36/1 -> GlobalConfig_Buscreator1/6  "Kp_n"
  Const22/1 -> Rate Transition45/1
  enableOnlineID1/1 -> Rate Transition53/1
  Const23/1 -> Rate Transition46/1
  Rate Transition60/1 -> Data Type Conversion53/1
  Const17/1 -> Rate Transition40/1
  2/1 -> Rate Transition60/1

== system uz_ParameterID6ph/dqTrans ==
  In Bus Element8 : Inport  PortName=ActualValues
  In Bus Element3 : Inport  PortName=ActualValues  Element=omega_el
  In Bus Element4 : Inport  PortName=ActualValues  Element=theta_m
  In Bus Element : Inport  PortName=ActualValues  Element=V_abc.a
  In Bus Element1 : Inport  PortName=ActualValues  Element=V_abc.b
  In Bus Element2 : Inport  PortName=ActualValues  Element=V_abc.c
  In Bus Element5 : Inport  PortName=ActualValues  Element=I_abc.a
  In Bus Element6 : Inport  PortName=ActualValues  Element=I_abc.b
  In Bus Element7 : Inport  PortName=ActualValues  Element=I_abc.c
  Bus Assignment : BusAssignment  AssignedSignals=v_dq.d,v_dq.q,V_abc.a,V_abc.b,V_abc.c,i_dq.d,i_dq.q
  Demux1 : Demux  Outputs=3
  Gain8 : Gain  Gain=d_p  OutDataTypeStr=single
  Mux : Mux  Inputs=3
  Terminator : Terminator
  Terminator1 : Terminator
  VoltageTransformation : Subsystem
  abc to dq0 : spsabctodq0Lib/abc to dq0  Alignment=Aligned with phase A axis
  ActualValues_corr : Outport  OutDataTypeStr=Bus: uz_ParaID_ActualValues_t
  wires:
  VoltageTransformation/3(0) -> Terminator1/1
  In Bus Element3/1 -> VoltageTransformation/4(omega_el)  "omega_m*polePairs"
  In Bus Element2/1 -> VoltageTransformation/3(u_c)  "u_c"
  In Bus Element1/1 -> VoltageTransformation/2(u_b)  "u_b"
  In Bus Element/1 -> VoltageTransformation/1(u_a)  "u_a"
  Demux1/3 -> Terminator/1
  Mux/1 -> abc to dq0/1
  In Bus Element7/1 -> Mux/3  "i_c"
  In Bus Element6/1 -> Mux/2  "i_b"
  In Bus Element5/1 -> Mux/1  "i_a"
  Demux1/2 -> Bus Assignment/8
  Demux1/1 -> Bus Assignment/7
  abc to dq0/1 -> Demux1/1
  VoltageTransformation/2(u_q) -> Bus Assignment/3
  VoltageTransformation/1(u_d) -> Bus Assignment/2
  VoltageTransformation/4(u_a_corr) -> Bus Assignment/4
  VoltageTransformation/5(u_b_corr) -> Bus Assignment/5
  VoltageTransformation/6(u_c_corr) -> Bus Assignment/6
  In Bus Element8/1 -> Bus Assignment/1
  Bus Assignment/1 -> ActualValues_corr/1
  Gain8/1 -> abc to dq0/2, VoltageTransformation/5(theta_el)  "theta_el"
  In Bus Element4/1 -> Gain8/1  "theta_m"

== system uz_ParameterID6ph/dqTrans1 ==
  In Bus Element8 : Inport  PortName=ActualValues
  In Bus Element9 : Inport  PortName=ActualValues  Element=V_abc.a1
  In Bus Element10 : Inport  PortName=ActualValues  Element=V_abc.b1
  In Bus Element11 : Inport  PortName=ActualValues  Element=V_abc.c1
  In Bus Element12 : Inport  PortName=ActualValues  Element=V_abc.a2
  In Bus Element13 : Inport  PortName=ActualValues  Element=V_abc.b2
  In Bus Element14 : Inport  PortName=ActualValues  Element=V_abc.c2
  In Bus Element1 : Inport  PortName=ActualValues  Element=I_abc.a1
  In Bus Element2 : Inport  PortName=ActualValues  Element=I_abc.b1
  In Bus Element3 : Inport  PortName=ActualValues  Element=I_abc.c1
  In Bus Element4 : Inport  PortName=ActualValues  Element=I_abc.a2
  In Bus Element16 : Inport  PortName=ActualValues  Element=I_abc.b2
  In Bus Element17 : Inport  PortName=ActualValues  Element=I_abc.c2
  In Bus Element15 : Inport  PortName=ActualValues  Element=theta_el
  In Bus Element18 : Inport  PortName=ActualValues  Element=theta_el
  Bus Assignment : BusAssignment  AssignedSignals=v_dq,i_dq
  Bus Creator : BusCreator  Inputs=6  OutDataTypeStr=Bus: uz_6ph_dq_t
  Bus Creator1 : BusCreator  Inputs=6  OutDataTypeStr=Bus: uz_6ph_dq_t
  Subsystem : Subsystem
  Subsystem1 : Subsystem
  ActualValues_corr : Outport  OutDataTypeStr=Bus: uz_ParaID6ph_ActualValues_t
  wires:
  In Bus Element8/1 -> Bus Assignment/1
  In Bus Element9/1 -> Subsystem/1(in_a1)
  In Bus Element10/1 -> Subsystem/2(in_b1)
  In Bus Element11/1 -> Subsystem/3(in_c1)
  In Bus Element14/1 -> Subsystem/6(in_c2)
  In Bus Element13/1 -> Subsystem/5(in_b2)
  In Bus Element12/1 -> Subsystem/4(in_a2)
  In Bus Element15/1 -> Subsystem/7(theta)  "theta_m"
  In Bus Element18/1 -> Subsystem1/7(theta)  "theta_m"
  In Bus Element4/1 -> Subsystem1/4(in_a2)
  In Bus Element16/1 -> Subsystem1/5(in_b2)
  In Bus Element17/1 -> Subsystem1/6(in_c2)
  In Bus Element3/1 -> Subsystem1/3(in_c1)
  In Bus Element2/1 -> Subsystem1/2(in_b1)
  In Bus Element1/1 -> Subsystem1/1(in_a1)
  Subsystem/6(out_z-) -> Bus Creator/6  "z2"
  Subsystem/5(out_z+) -> Bus Creator/5  "z1"
  Subsystem/4(out_y) -> Bus Creator/4  "y"
  Subsystem/3(out_x) -> Bus Creator/3  "x"
  Subsystem/2(out_q) -> Bus Creator/2  "q"
  Subsystem/1(out_d) -> Bus Creator/1  "d"
  Subsystem1/1(out_d) -> Bus Creator1/1  "d"
  Subsystem1/2(out_q) -> Bus Creator1/2  "q"
  Subsystem1/3(out_x) -> Bus Creator1/3  "x"
  Subsystem1/4(out_y) -> Bus Creator1/4  "y"
  Subsystem1/5(out_z+) -> Bus Creator1/5  "z1"
  Subsystem1/6(out_z-) -> Bus Creator1/6  "z2"
  Bus Creator/1 -> Bus Assignment/2
  Bus Creator1/1 -> Bus Assignment/3
  Bus Assignment/1 -> ActualValues_corr/1

== system uz_ParameterID6ph/FOC/PWM Generator ==
  Bus Element In2 : Inport  PortName=ActualValues  Element=theta_m
  Bus Element In3 : Inport  PortName=ActualValues  Element=V_DC
  v_dq_ref : Inport  Port=2
  Constant : Constant  OutDataTypeStr=single
  Constant1 : Constant  Value=0  OutDataTypeStr=single
  Demux1 : Demux  Outputs=2
  Demux2 : Demux  Outputs=3
  Divide3 : Product  Inputs=*/
  Gain : Gain  Gain=0.5
  Gain4 : Gain  Gain=0.5
  Gain8 : Gain  Gain=d_p  OutDataTypeStr=single
  Mux1 : Mux  Inputs=3
  Saturation2 : Saturate  UpperLimit=1  LowerLimit=0
  Scope3 : Scope  NumInputPorts=3
  Sum5 : Sum  Inputs=|++
  dq0 to abc : spsdq0toabcLib/dq0 to abc  Alignment=Aligned with phase A axis
  PWM_024_out : Outport  VectorParamsAs1DForOutWhenUnconnected=off
  wires:
  Constant/1 -> Sum5/2
  Demux2/2 -> Scope3/2
  Gain4/1 -> Saturation2/1
  Demux2/1 -> Scope3/1
  Demux2/3 -> Scope3/3
  Gain/1 -> Divide3/2
  Sum5/1 -> Gain4/1
  Mux1/1 -> dq0 to abc/1
  dq0 to abc/1 -> Demux2/1, Divide3/1
  Divide3/1 -> Sum5/1
  Bus Element In3/1 -> Gain/1
  Constant1/1 -> Mux1/3
  Demux1/2 -> Mux1/2
  Saturation2/1 -> PWM_024_out/1
  v_dq_ref/1 -> Demux1/1
  Demux1/1 -> Mux1/1
  Bus Element In2/1 -> Gain8/1
  Gain8/1 -> dq0 to abc/2  "theta_el"

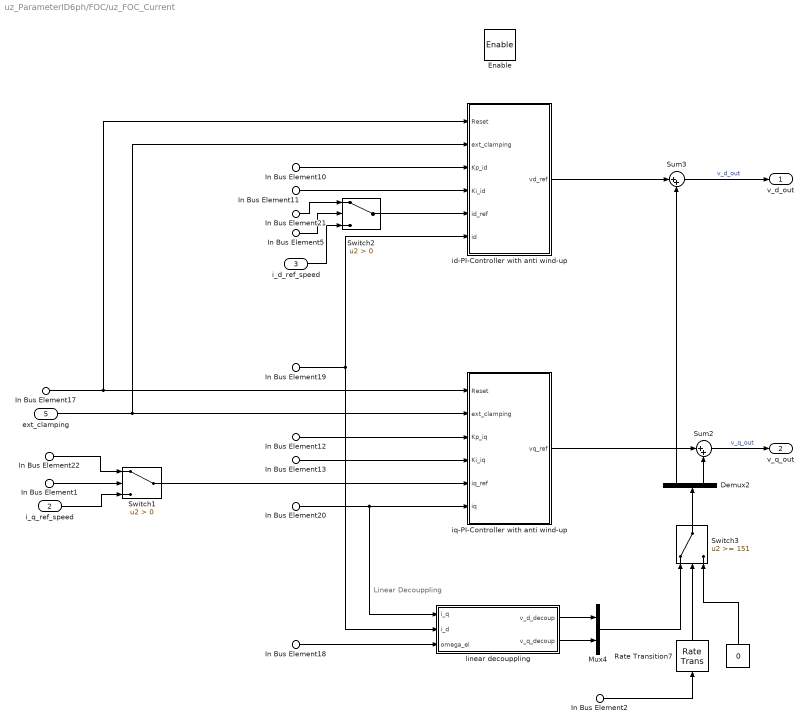
== system uz_ParameterID6ph/FOC/uz_FOC_Current ==
  note: Linear Decouppling
  In Bus Element18 : Inport  PortName=ActualValues  Element=omega_el
  In Bus Element19 : Inport  PortName=ActualValues  Element=i_dq.d
  In Bus Element20 : Inport  PortName=ActualValues  Element=i_dq.q
  i_q_ref_speed : Inport  Port=2
  i_d_ref_speed : Inport  Port=3
  In Bus Element17 : Inport  Port=4  PortName=FOC_State_outputs  Element=resetIntegrator
  In Bus Element11 : Inport  Port=4  PortName=FOC_State_outputs  Element=Ki_id_out
  In Bus Element10 : Inport  Port=4  PortName=FOC_State_outputs  Element=Kp_id_out
  In Bus Element12 : Inport  Port=4  PortName=FOC_State_outputs  Element=Kp_iq_out
  In Bus Element13 : Inport  Port=4  PortName=FOC_State_outputs  Element=Ki_iq_out
  In Bus Element1 : Inport  Port=4  PortName=FOC_State_outputs  Element=enableFOC_current
  In Bus Element5 : Inport  Port=4  PortName=FOC_State_outputs  Element=enableFOC_current
  In Bus Element2 : Inport  Port=4  PortName=FOC_State_outputs  Element=activeState
  In Bus Element21 : Inport  Port=4  PortName=FOC_State_outputs  Element=i_dq_ref.d
  In Bus Element22 : Inport  Port=4  PortName=FOC_State_outputs  Element=i_dq_ref.q
  ext_clamping : Inport  Port=5
  Enable : EnablePort
  " " : Constant  Value=0  OutDataTypeStr=single
  Demux2 : Demux  Outputs=2
  Mux4 : Mux  Inputs=2
  Rate Transition7 : RateTransition  OutPortSampleTime=1/d_f_hardware
  Sum2 : Sum  Inputs=|++
  Sum3 : Sum  Inputs=|++
  Switch1 : Switch  Criteria=u2 > Threshold
  Switch2 : Switch  Criteria=u2 > Threshold
  Switch3 : Switch  Threshold=151
  id-PI-Controller with anti wind-up : Subsystem
  iq-PI-Controller with anti wind-up : Subsystem
  linear decouppling : Subsystem
  v_d_out : Outport
  v_q_out : Outport  Port=2
  wires:
  In Bus Element22/1 -> Switch1/1
  In Bus Element1/1 -> Switch1/2
  Demux2/2 -> Sum2/2
  id-PI-Controller with anti wind-up/1(vd_ref) -> Sum3/1
  In Bus Element19/1 -> id-PI-Controller with anti wind-up/6(id), linear decouppling/2(i_d)
  Demux2/1 -> Sum3/2
  linear decouppling/2(v_q_decoup) -> Mux4/2
  linear decouppling/1(v_d_decoup) -> Mux4/1
  ext_clamping/1 -> iq-PI-Controller with anti wind-up/2(ext_clamping), id-PI-Controller with anti wind-up/2(ext_clamping)
  Switch1/1 -> iq-PI-Controller with anti wind-up/5(iq_ref)
  Sum3/1 -> v_d_out/1  "v_d_out"
  In Bus Element10/1 -> id-PI-Controller with anti wind-up/3(Kp_id)
  In Bus Element18/1 -> linear decouppling/3(omega_el)
  In Bus Element17/1 -> iq-PI-Controller with anti wind-up/1(Reset), id-PI-Controller with anti wind-up/1(Reset)
  In Bus Element12/1 -> iq-PI-Controller with anti wind-up/3(Kp_iq)
  i_q_ref_speed/1 -> Switch1/3
  iq-PI-Controller with anti wind-up/1(vq_ref) -> Sum2/1
  In Bus Element20/1 -> linear decouppling/1(i_q), iq-PI-Controller with anti wind-up/6(iq)
  i_d_ref_speed/1 -> Switch2/3
  In Bus Element21/1 -> Switch2/1
  Switch2/1 -> id-PI-Controller with anti wind-up/5(id_ref)
  In Bus Element5/1 -> Switch2/2
  Mux4/1 -> Switch3/1
  In Bus Element13/1 -> iq-PI-Controller with anti wind-up/4(Ki_iq)
  In Bus Element11/1 -> id-PI-Controller with anti wind-up/4(Ki_id)
  Sum2/1 -> v_q_out/1  "v_q_out"
  In Bus Element2/1 -> Rate Transition7/1
  Rate Transition7/1 -> Switch3/2
  Switch3/1 -> Demux2/1
  " "/1 -> Switch3/3

== system uz_ParameterID6ph/FOC/uz_FOC_Speed ==
  In Bus Element18 : Inport  PortName=ActualValues  Element=omega_el
  In Bus Element19 : Inport  PortName=ActualValues  Element=V_DC
  In Bus Element : Inport  Port=2  PortName=TwoMassID_output  Element=PRBS_out
  In Bus Element13 : Inport  Port=3  PortName=FOC_State_outputs  Element=Kp_n_out
  In Bus Element14 : Inport  Port=3  PortName=FOC_State_outputs  Element=Ki_n_out
  In Bus Element15 : Inport  Port=3  PortName=FOC_State_outputs  Element=n_ref_FOC
  In Bus Element5 : Inport  Port=3  PortName=FOC_State_outputs  Element=resetIntegrator
  In Bus Element21 : Inport  Port=3  PortName=FOC_State_outputs  Element=i_dq_ref.d
  ext_clamping : Inport  Port=4
  Enable : EnablePort
  Field Weakening : Subsystem
  Sum5 : Sum  Inputs=|++
  omega-PI-Controller with anti wind-up : Subsystem
  i_q_ref : Outport  OutDataTypeStr=single
  id_soll : Outport  Port=2  OutDataTypeStr=single
  wires:
  In Bus Element/1 -> Sum5/2  "PRBS Excitation"
  In Bus Element21/1 -> Field Weakening/3(id_ref_input)
  In Bus Element13/1 -> omega-PI-Controller with anti wind-up/3(Kp_n)
  Field Weakening/2(id_Soll) -> id_soll/1
  In Bus Element19/1 -> Field Weakening/2(V_DC)
  ext_clamping/1 -> omega-PI-Controller with anti wind-up/2(ext_clamping)
  In Bus Element18/1 -> Field Weakening/1(omega_el), omega-PI-Controller with anti wind-up/6(omega)
  In Bus Element14/1 -> omega-PI-Controller with anti wind-up/4(Ki_n)
  In Bus Element15/1 -> omega-PI-Controller with anti wind-up/5(n_ref_rpm)
  In Bus Element5/1 -> omega-PI-Controller with anti wind-up/1(Reset)
  omega-PI-Controller with anti wind-up/1(iq_ref) -> Sum5/1
  Sum5/1 -> i_q_ref/1
  Field Weakening/1(iq_max) -> omega-PI-Controller with anti wind-up/7(iq_max)

== system uz_ParameterID6ph/Hardware/Coupling Encoder ==
  note: 1) Add Subsystem or Model blocks as valid variant choices.
      | 2) You cannot connect blocks at this level. At simulation, connectivity is automatically
      | determined, based on the active variant and port name matching.
  Inertia : Subsystem  VariantControl=(default)
  Spring Damper System : Subsystem  VariantControl=TMS1
  Input : PMIOPort  Side=Left
  output : PMIOPort  Port=2  Side=Right

== system uz_ParameterID6ph/Hardware/Measurement Shaft ==
  note: 1) Add Subsystem or Model blocks as valid variant choices.
      | 2) You cannot connect blocks at this level. At simulation, connectivity is automatically
      | determined, based on the active variant and port name matching.
  Spring Damper System : Subsystem  VariantControl=TMS1
  default : Subsystem  VariantControl=(default)
  Input : PMIOPort  Side=Left
  output : PMIOPort  Port=2  Side=Right

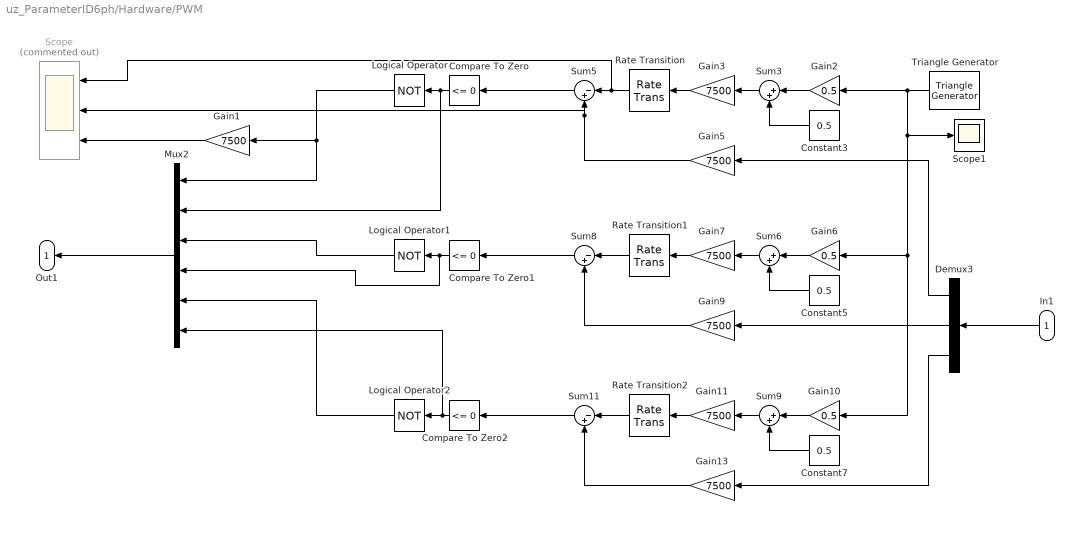
== system uz_ParameterID6ph/Hardware/PWM ==
  In1 : Inport
  Compare To Zero : simulink/Logic and Bit Operations/Compare To Zero  relop=<=  OutDataTypeStr=boolean
  Compare To Zero1 : simulink/Logic and Bit Operations/Compare To Zero  relop=<=  OutDataTypeStr=boolean
  Compare To Zero2 : simulink/Logic and Bit Operations/Compare To Zero  relop=<=  OutDataTypeStr=boolean
  Constant3 : Constant  Value=0.5
  Constant5 : Constant  Value=0.5
  Constant7 : Constant  Value=0.5
  Demux3 : Demux  Outputs=3
  Gain{1,3,5,7,9,11,13} (7 alike) : Gain  Gain=7500  ParamDataTypeStr=single
  Gain10 : Gain  Gain=0.5
  Gain2 : Gain  Gain=0.5
  Gain6 : Gain  Gain=0.5
  Logical Operator : Logic  Operator=NOT  AllPortsSameDT=off  OutDataTypeStr=boolean
  Logical Operator1 : Logic  Operator=NOT  AllPortsSameDT=off  OutDataTypeStr=boolean
  Logical Operator2 : Logic  Operator=NOT  AllPortsSameDT=off  OutDataTypeStr=boolean
  Mux2 : Mux  Inputs=6
  Rate Transition : RateTransition  OutPortSampleTime=1/d_f_hardware
  Rate Transition1 : RateTransition  OutPortSampleTime=1/d_f_hardware
  Rate Transition2 : RateTransition  OutPortSampleTime=1/d_f_hardware
  Scope : Scope  Commented=on  NumInputPorts=3
  Scope1 : Scope
  Sum11 : Sum  Inputs=|-+
  Sum3 : Sum  Inputs=|++
  Sum5 : Sum  Inputs=|-+
  Sum6 : Sum  Inputs=|++
  Sum8 : Sum  Inputs=|-+
  Sum9 : Sum  Inputs=|++
  Triangle Generator : spsTriangleGeneratorLib/Triangle Generator  Freq=10000  Phase=0  Ts=0
  Out1 : Outport  VectorParamsAs1DForOutWhenUnconnected=off
  wires:
  Demux3/3 -> Gain13/1
  Logical Operator2/1 -> Mux2/5
  Logical Operator1/1 -> Mux2/3
  Mux2/1 -> Out1/1
  Compare To Zero2/1 -> Mux2/6, Logical Operator2/1
  Gain10/1 -> Sum9/1
  Sum8/1 -> Compare To Zero1/1
  Gain6/1 -> Sum6/1
  Sum9/1 -> Gain11/1
  Triangle Generator/1 -> Scope1/1, Gain10/1, Gain6/1, Gain2/1
  Sum6/1 -> Gain7/1
  Demux3/2 -> Gain9/1
  Compare To Zero1/1 -> Mux2/4, Logical Operator1/1
  Constant5/1 -> Sum6/2
  Constant7/1 -> Sum9/2
  Sum11/1 -> Compare To Zero2/1
  Sum3/1 -> Gain3/1
  Constant3/1 -> Sum3/2
  Demux3/1 -> Gain5/1
  Sum5/1 -> Compare To Zero/1
  Gain2/1 -> Sum3/1
  In1/1 -> Demux3/1
  Gain3/1 -> Rate Transition/1
  Gain7/1 -> Rate Transition1/1
  Gain11/1 -> Rate Transition2/1
  Gain5/1 -> Scope/2, Sum5/2
  Gain9/1 -> Sum8/2
  Gain13/1 -> Sum11/2
  Rate Transition/1 -> Scope/1, Sum5/1
  Rate Transition1/1 -> Sum8/1
  Rate Transition2/1 -> Sum11/1
  Logical Operator/1 -> Gain1/1, Mux2/1
  Compare To Zero/1 -> Mux2/2, Logical Operator/1
  Gain1/1 -> Scope/3

== system uz_ParameterID6ph/Hardware/Switch f. TMS ==
  note: 1) Add Subsystem or Model blocks as valid variant choices.
      | 2) You cannot connect blocks at this level. At simulation, connectivity is automatically
      | determined, based on the active variant and port name matching.
  closed : Subsystem  VariantControl=d_KupplZus==1
  open : Subsystem  VariantControl=d_KupplZus==0
  Input : PMIOPort  Side=Left
  output : PMIOPort  Port=2  Side=Right

== system uz_ParameterID6ph/Hardware/coupling m. shaft ==
  note: 1) Add Subsystem or Model blocks as valid variant choices.
      | 2) You cannot connect blocks at this level. At simulation, connectivity is automatically
      | determined, based on the active variant and port name matching.
  Inertia : Subsystem  VariantControl=(default)
  Spring Damper System : Subsystem  VariantControl=TMS1
  Input : PMIOPort  Side=Left
  output : PMIOPort  Port=2  Side=Right

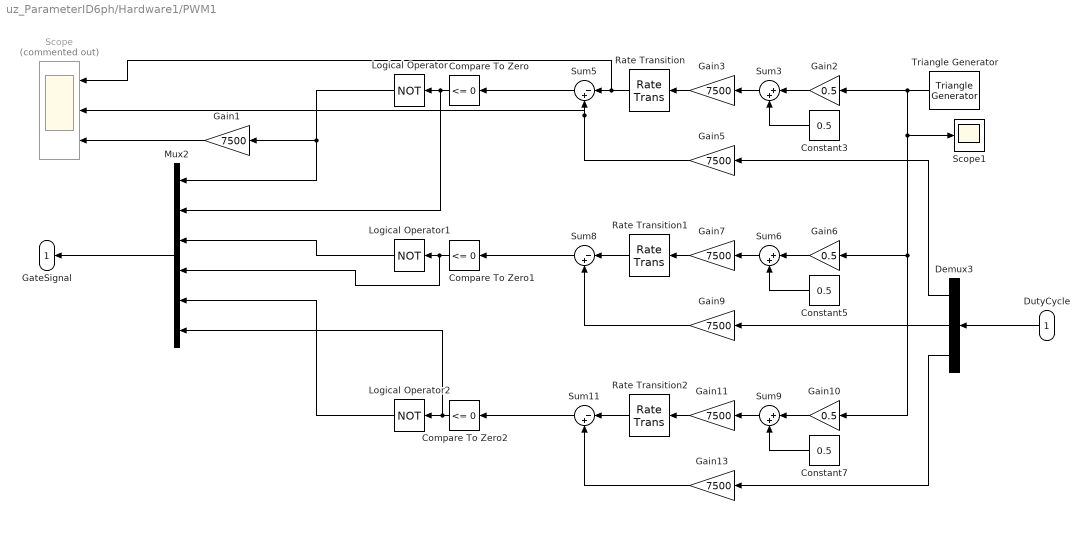
== system uz_ParameterID6ph/Hardware1/PWM1 ==
  DutyCycle : Inport
  Compare To Zero : simulink/Logic and Bit Operations/Compare To Zero  relop=<=  OutDataTypeStr=boolean
  Compare To Zero1 : simulink/Logic and Bit Operations/Compare To Zero  relop=<=  OutDataTypeStr=boolean
  Compare To Zero2 : simulink/Logic and Bit Operations/Compare To Zero  relop=<=  OutDataTypeStr=boolean
  Constant3 : Constant  Value=0.5
  Constant5 : Constant  Value=0.5
  Constant7 : Constant  Value=0.5
  Demux3 : Demux  Outputs=3
  Gain{1,3,5,7,9,11,13} (7 alike) : Gain  Gain=7500  ParamDataTypeStr=single
  Gain10 : Gain  Gain=0.5
  Gain2 : Gain  Gain=0.5
  Gain6 : Gain  Gain=0.5
  Logical Operator : Logic  Operator=NOT  AllPortsSameDT=off  OutDataTypeStr=boolean
  Logical Operator1 : Logic  Operator=NOT  AllPortsSameDT=off  OutDataTypeStr=boolean
  Logical Operator2 : Logic  Operator=NOT  AllPortsSameDT=off  OutDataTypeStr=boolean
  Mux2 : Mux  Inputs=6
  Rate Transition : RateTransition  OutPortSampleTime=1/d_f_hardware
  Rate Transition1 : RateTransition  OutPortSampleTime=1/d_f_hardware
  Rate Transition2 : RateTransition  OutPortSampleTime=1/d_f_hardware
  Scope : Scope  Commented=on  NumInputPorts=3
  Scope1 : Scope
  Sum11 : Sum  Inputs=|-+
  Sum3 : Sum  Inputs=|++
  Sum5 : Sum  Inputs=|-+
  Sum6 : Sum  Inputs=|++
  Sum8 : Sum  Inputs=|-+
  Sum9 : Sum  Inputs=|++
  Triangle Generator : spsTriangleGeneratorLib/Triangle Generator  Freq=10000  Phase=0  Ts=0
  GateSignal : Outport  VectorParamsAs1DForOutWhenUnconnected=off
  wires:
  Demux3/3 -> Gain13/1
  Logical Operator2/1 -> Mux2/5
  Logical Operator1/1 -> Mux2/3
  Mux2/1 -> GateSignal/1
  Compare To Zero2/1 -> Mux2/6, Logical Operator2/1
  Gain10/1 -> Sum9/1
  Sum8/1 -> Compare To Zero1/1
  Gain6/1 -> Sum6/1
  Sum9/1 -> Gain11/1
  Triangle Generator/1 -> Scope1/1, Gain10/1, Gain6/1, Gain2/1
  Sum6/1 -> Gain7/1
  Demux3/2 -> Gain9/1
  Compare To Zero1/1 -> Mux2/4, Logical Operator1/1
  Constant5/1 -> Sum6/2
  Constant7/1 -> Sum9/2
  Sum11/1 -> Compare To Zero2/1
  Sum3/1 -> Gain3/1
  Constant3/1 -> Sum3/2
  Demux3/1 -> Gain5/1
  Sum5/1 -> Compare To Zero/1
  Gain2/1 -> Sum3/1
  DutyCycle/1 -> Demux3/1
  Gain3/1 -> Rate Transition/1
  Gain7/1 -> Rate Transition1/1
  Gain11/1 -> Rate Transition2/1
  Gain5/1 -> Scope/2, Sum5/2
  Gain9/1 -> Sum8/2
  Gain13/1 -> Sum11/2
  Rate Transition/1 -> Scope/1, Sum5/1
  Rate Transition1/1 -> Sum8/1
  Rate Transition2/1 -> Sum11/1
  Logical Operator/1 -> Gain1/1, Mux2/1
  Compare To Zero/1 -> Mux2/2, Logical Operator/1
  Gain1/1 -> Scope/3

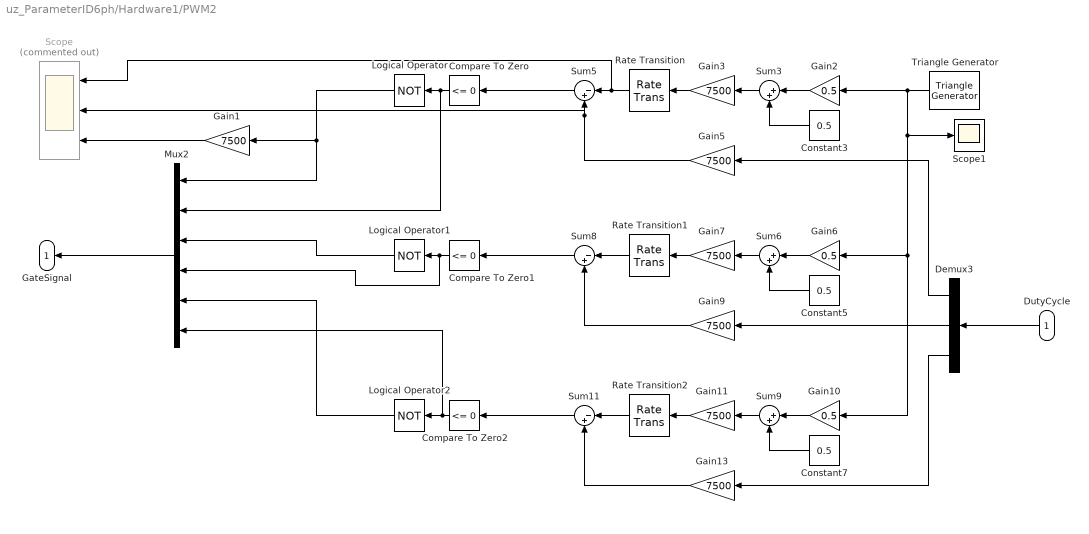
== system uz_ParameterID6ph/Hardware1/PWM2 ==
  DutyCycle : Inport
  Compare To Zero : simulink/Logic and Bit Operations/Compare To Zero  relop=<=  OutDataTypeStr=boolean
  Compare To Zero1 : simulink/Logic and Bit Operations/Compare To Zero  relop=<=  OutDataTypeStr=boolean
  Compare To Zero2 : simulink/Logic and Bit Operations/Compare To Zero  relop=<=  OutDataTypeStr=boolean
  Constant3 : Constant  Value=0.5
  Constant5 : Constant  Value=0.5
  Constant7 : Constant  Value=0.5
  Demux3 : Demux  Outputs=3
  Gain{1,3,5,7,9,11,13} (7 alike) : Gain  Gain=7500  ParamDataTypeStr=single
  Gain10 : Gain  Gain=0.5
  Gain2 : Gain  Gain=0.5
  Gain6 : Gain  Gain=0.5
  Logical Operator : Logic  Operator=NOT  AllPortsSameDT=off  OutDataTypeStr=boolean
  Logical Operator1 : Logic  Operator=NOT  AllPortsSameDT=off  OutDataTypeStr=boolean
  Logical Operator2 : Logic  Operator=NOT  AllPortsSameDT=off  OutDataTypeStr=boolean
  Mux2 : Mux  Inputs=6
  Rate Transition : RateTransition  OutPortSampleTime=1/d_f_hardware
  Rate Transition1 : RateTransition  OutPortSampleTime=1/d_f_hardware
  Rate Transition2 : RateTransition  OutPortSampleTime=1/d_f_hardware
  Scope : Scope  Commented=on  NumInputPorts=3
  Scope1 : Scope
  Sum11 : Sum  Inputs=|-+
  Sum3 : Sum  Inputs=|++
  Sum5 : Sum  Inputs=|-+
  Sum6 : Sum  Inputs=|++
  Sum8 : Sum  Inputs=|-+
  Sum9 : Sum  Inputs=|++
  Triangle Generator : spsTriangleGeneratorLib/Triangle Generator  Freq=10000  Phase=0  Ts=0
  GateSignal : Outport  VectorParamsAs1DForOutWhenUnconnected=off
  wires:
  Gain1/1 -> Scope/3
  Compare To Zero/1 -> Logical Operator/1, Mux2/2
  Logical Operator/1 -> Mux2/1, Gain1/1
  Rate Transition2/1 -> Sum11/1
  Rate Transition1/1 -> Sum8/1
  Rate Transition/1 -> Sum5/1, Scope/1
  Gain13/1 -> Sum11/2
  Gain9/1 -> Sum8/2
  Gain5/1 -> Sum5/2, Scope/2
  Gain11/1 -> Rate Transition2/1
  Gain7/1 -> Rate Transition1/1
  Gain3/1 -> Rate Transition/1
  DutyCycle/1 -> Demux3/1
  Gain2/1 -> Sum3/1
  Sum5/1 -> Compare To Zero/1
  Demux3/1 -> Gain5/1
  Constant3/1 -> Sum3/2
  Sum3/1 -> Gain3/1
  Sum11/1 -> Compare To Zero2/1
  Constant7/1 -> Sum9/2
  Constant5/1 -> Sum6/2
  Compare To Zero1/1 -> Logical Operator1/1, Mux2/4
  Demux3/2 -> Gain9/1
  Sum6/1 -> Gain7/1
  Triangle Generator/1 -> Gain2/1, Gain6/1, Gain10/1, Scope1/1
  Sum9/1 -> Gain11/1
  Gain6/1 -> Sum6/1
  Sum8/1 -> Compare To Zero1/1
  Gain10/1 -> Sum9/1
  Compare To Zero2/1 -> Logical Operator2/1, Mux2/6
  Mux2/1 -> GateSignal/1
  Logical Operator1/1 -> Mux2/3
  Logical Operator2/1 -> Mux2/5
  Demux3/3 -> Gain13/1
